simulink model "interpolation_nD_TestGen34"  (R2017b)
settings: Solver=FixedStepDiscrete  StartTime=0.0  StopTime=10.0  RelTol=1e-3
PreLoadFcn:
  |  LUTObj = Simulink.LookupTable;
  |  LUTObj.Table.Value = [29.1117932179652 28.5374745197584;99.2404976402485 112.371519326068;122.533671431908 120.247876884759];
  |  LUTObj.Table.DataType = 'auto';
  |  LUTObj.StructTypeInfo.Name = 'myLUTStruct';
  |  LUTObj.BreakpointsSpecification = 'Reference';
  |  LUTObj.Breakpoints{1} = 'myBpSet1';
  | myBpSet1 = Simulink.Breakpoint;
  | myBpSet1.Breakpoints.Value = [1 2 3];
  |  LUTObj.Breakpoints{2} = 'myBpSet2';
  | myBpSet2 = Simulink.Breakpoint;
  | myBpSet2.Breakpoints.Value = [1 2];
settings Model: Creator=ktrinh  LastModifiedBy=ktrinh
settings DebuggingCC: ParameterOverflowMsg=none

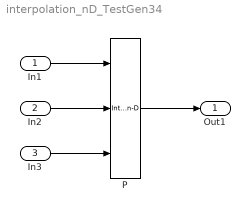
== system interpolation_nD_TestGen34 ==
  In1 : Inport  OutMin=0  OutMax=3  PortDimensions=[2,3]
  In2 : Inport  Port=2  OutMin=-0.5  OutMax=1.5
  In3 : Inport  Port=3  OutMin=0  OutMax=2
  P : Interpolation_n-D  Table=[29.1117932179652 28.5374745197584;99.2404976402485 112.371519326068;122.533671431908 120.247876884759]  TableSpecification=Lookup table object  LookupTableObject=LUTObj  InterpMethod=Nearest  NumSelectionDims=1  OutDataTypeStr=int8  InternalRulePriority=Speed  RndMeth=Zero
      settings: InputPortMap=u0,u1,u2
  Out1 : Outport
  wires:
  In1/1 -> P/1
  In2/1 -> P/2
  In3/1 -> P/3
  P/1 -> Out1/1
